simulink model "conv_kernel_2019b"  (R2019b)
settings: Solver=VariableStepAuto  StartTime=0.0  StopTime=2  RelTol=1e-3
values from neighbouring files (symbols this model uses):
  RGB = 1    [setup.m]
  rgb_limits = [r_min g_min b_min ... (first row only)    [setup.m]
  Ts = 1    [setup.m]
  YCbCr = 0    [setup.m]
  YCbCr_limits = [y_min cb_min cr_min ... (first row only)    [setup.m]
undefined symbols (not defined in the file or in its folder): Rec, SDTV
libraries: visionconversions x1, visionsources x1
settings Model: Creator=David  LastModifiedBy=David

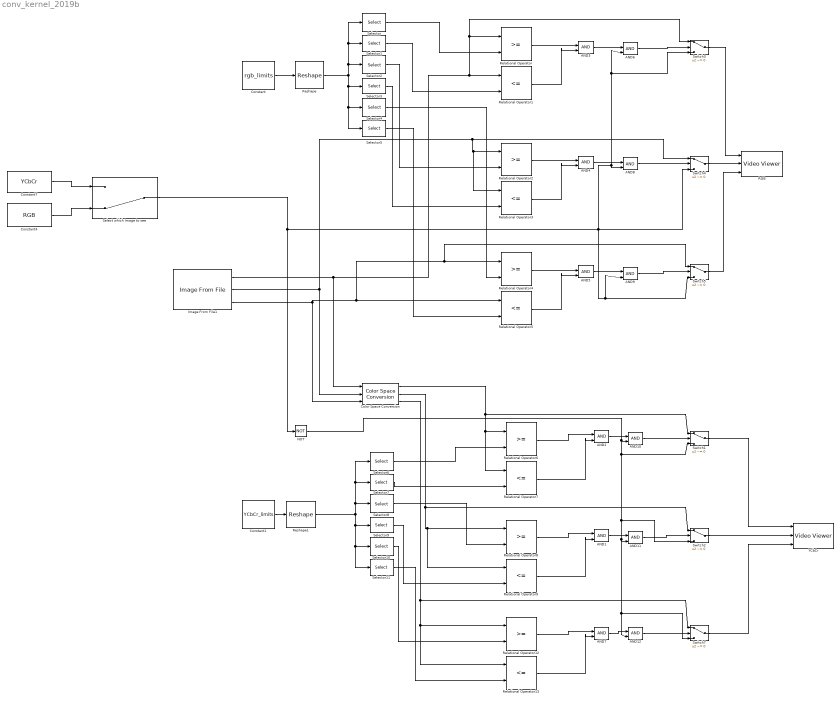
== system conv_kernel_2019b ==
  AND{1..12} (12 alike) : Logic  IconShape=distinctive  AllPortsSameDT=off  OutDataTypeStr=boolean
  Color Space Conversion : visionconversions/Color Space  Conversion  conversion=Obsolete  conversionActive=R'G'B' to Y'CbCr  wp_str=D65  rec=Rec. 601 (SDTV)  sys=1125/60/2:1  imagePorts=Separate color signals
  Constant : Constant  Value=rgb_limits  SampleTime=Ts
  Constant1 : Constant  Value=YCbCr_limits  SampleTime=Ts
  Constant4 : Constant  Value=RGB  SampleTime=Ts
  Constant7 : Constant  Value=YCbCr  SampleTime=Ts
  Image From File1 : visionsources/Image From File  Tag=vipblks_nd  FileName=sailboat.jpg  Ts=Ts  imagePorts=Separate color signals  OutPortLabels=R|G|B  ImageDataType=Inherit from input image  sdImageDataType=uint(8)  Signed=on  WordLength=16  FractionLengthMode=User-defined  FractionLength=15
  NOT : Logic  Operator=NOT  IconShape=distinctive  AllPortsSameDT=off  OutDataTypeStr=boolean
  RGB : VideoViewer  imagePorts=separate color signals  FigPos=[1337 969 858 742]
  Relational Operator{,2,4,6,8,12} (6 alike) : RelationalOperator  OutDataTypeStr=boolean  RndMeth=Simplest
  Relational Operator{1,3,5,7,9,13} (6 alike) : RelationalOperator  Operator=<=  OutDataTypeStr=boolean  RndMeth=Simplest
  Reshape : Reshape
  Reshape1 : Reshape
  Select which Image to see : ManualSwitch  CurrentSetting=0
  Selector : Selector  IndexMode=Zero-based  InputPortWidth=6  IndexOptions=Index vector (dialog)  Indices=0  OutputSizes=2
  Selector1 : Selector  IndexMode=Zero-based  InputPortWidth=6  IndexOptions=Index vector (dialog)  Indices=1  OutputSizes=1
  Selector10 : Selector  IndexMode=Zero-based  InputPortWidth=6  IndexOptions=Index vector (dialog)  Indices=4  OutputSizes=1
  Selector11 : Selector  IndexMode=Zero-based  InputPortWidth=6  IndexOptions=Index vector (dialog)  Indices=5  OutputSizes=1
  Selector2 : Selector  IndexMode=Zero-based  InputPortWidth=6  IndexOptions=Index vector (dialog)  Indices=2  OutputSizes=1
  Selector3 : Selector  IndexMode=Zero-based  InputPortWidth=6  IndexOptions=Index vector (dialog)  Indices=3  OutputSizes=1
  Selector4 : Selector  IndexMode=Zero-based  InputPortWidth=6  IndexOptions=Index vector (dialog)  Indices=4  OutputSizes=1
  Selector5 : Selector  IndexMode=Zero-based  InputPortWidth=6  IndexOptions=Index vector (dialog)  Indices=5  OutputSizes=1
  Selector6 : Selector  IndexMode=Zero-based  InputPortWidth=6  IndexOptions=Index vector (dialog)  Indices=0  OutputSizes=2
  Selector7 : Selector  IndexMode=Zero-based  InputPortWidth=6  IndexOptions=Index vector (dialog)  Indices=1  OutputSizes=1
  Selector8 : Selector  IndexMode=Zero-based  InputPortWidth=6  IndexOptions=Index vector (dialog)  Indices=2  OutputSizes=1
  Selector9 : Selector  IndexMode=Zero-based  InputPortWidth=6  IndexOptions=Index vector (dialog)  Indices=3  OutputSizes=1
  Switch{1..5,7} (6 alike) : Switch  Criteria=u2 ~= 0  OutDataTypeStr=uint8
  YCbCr : VideoViewer  imagePorts=separate color signals  FigPos=[174 968 1135 745]
  wires:
  Image From File1/2 -> Relational Operator3/1, Relational Operator2/1, Switch4/1, Color Space Conversion/2
  Image From File1/3 -> Switch5/1, Relational Operator4/1, Relational Operator5/1, Color Space Conversion/3
  Constant/1 -> Reshape/1
  Reshape/1 -> Selector/1, Selector1/1, Selector2/1, Selector5/1, Selector4/1, Selector3/1
  Image From File1/1 -> Relational Operator1/1, Switch3/1, Relational Operator/1, Color Space Conversion/1
  Selector/1 -> Relational Operator/2
  Selector1/1 -> Relational Operator1/2
  Relational Operator/1 -> AND3/1
  Relational Operator1/1 -> AND3/2
  Switch3/1 -> RGB/1
  Relational Operator3/1 -> AND4/2
  Relational Operator2/1 -> AND4/1
  Selector2/1 -> Relational Operator2/2
  Selector3/1 -> Relational Operator3/2
  Switch5/1 -> RGB/3
  Relational Operator4/1 -> AND5/1
  Relational Operator5/1 -> AND5/2
  Selector4/1 -> Relational Operator4/2
  Selector5/1 -> Relational Operator5/2
  Switch4/1 -> RGB/2
  Reshape1/1 -> Selector6/1, Selector7/1, Selector8/1, Selector9/1, Selector10/1, Selector11/1
  Constant1/1 -> Reshape1/1
  Selector6/1 -> Relational Operator6/2
  Selector7/1 -> Relational Operator7/2
  Color Space Conversion/1 -> Relational Operator7/1, Relational Operator6/1, Switch1/1
  Relational Operator6/1 -> AND2/1
  Relational Operator7/1 -> AND2/2
  Switch1/1 -> YCbCr/1
  Relational Operator9/1 -> AND1/2
  Relational Operator8/1 -> AND1/1
  Color Space Conversion/2 -> Switch2/1, Relational Operator9/1, Relational Operator8/1
  Relational Operator13/1 -> AND7/2
  Relational Operator12/1 -> AND7/1
  Color Space Conversion/3 -> Relational Operator13/1, Relational Operator12/1, Switch7/1
  Selector8/1 -> Relational Operator8/2
  Selector9/1 -> Relational Operator9/2
  Selector10/1 -> Relational Operator12/2
  Selector11/1 -> Relational Operator13/2
  Switch2/1 -> YCbCr/2
  Switch7/1 -> YCbCr/3
  AND3/1 -> AND6/1
  Select which Image to see/1 -> NOT/1, AND9/2, Switch5/3, Switch3/3, AND6/2, AND8/2, Switch4/3
  AND6/1 -> Switch3/2
  AND4/1 -> AND8/1
  AND8/1 -> Switch4/2
  AND5/1 -> AND9/1
  AND9/1 -> Switch5/2
  Constant7/1 -> Select which Image to see/1
  Constant4/1 -> Select which Image to see/2
  AND2/1 -> AND10/1
  NOT/1 -> Switch2/3, Switch7/3, AND12/2, AND11/2, Switch1/3, AND10/2
  AND10/1 -> Switch1/2
  AND7/1 -> AND12/1
  AND1/1 -> AND11/1
  AND11/1 -> Switch2/2
  AND12/1 -> Switch7/2
